simulink subsystem "free_lift"  (R2020a)
settings: Solver=VariableStepAuto  StartTime=0.0  StopTime=10.0  RelTol=1e-3
settings Model: Creator=Philip  LastModifiedBy=Philip

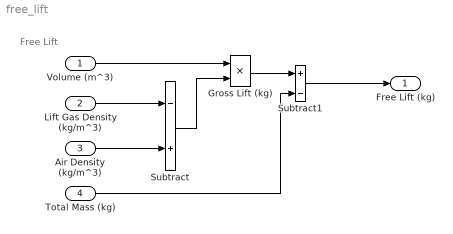
== system free_lift ==
  note: Free Lift
  Volume (m^3) : Inport
  Lift Gas Density (kg/m^3) : Inport  Port=2
  Air Density (kg/m^3) : Inport  Port=3
  Total Mass (kg) : Inport  Port=4
  Gross Lift (kg) : Product
  Subtract : Sum  Inputs=-+
  Subtract1 : Sum  Inputs=+-
  Free Lift (kg) : Outport
  wires:
  Air Density (kg/m^3)/1 -> Subtract/2
  Lift Gas Density (kg/m^3)/1 -> Subtract/1
  Volume (m^3)/1 -> Gross Lift (kg)/1
  Subtract/1 -> Gross Lift (kg)/2
  Gross Lift (kg)/1 -> Subtract1/1
  Total Mass (kg)/1 -> Subtract1/2
  Subtract1/1 -> Free Lift (kg)/1
